simulink model "Maglev_sim_2"  (R2024b)
settings: Solver=ode23tb  StartTime=0.0  StopTime=15  MaxStep=1e-3  RelTol=1e-3
undefined symbols (not defined in the file): A, A0, A0_obv, Adj, B, B0, B0_obv, c, C, C0, C0_obv, D, D0, D0_obv, F, G, K, K0
libraries: simulink x4
settings Model: Creator=coron  LastModifiedBy=rgivo

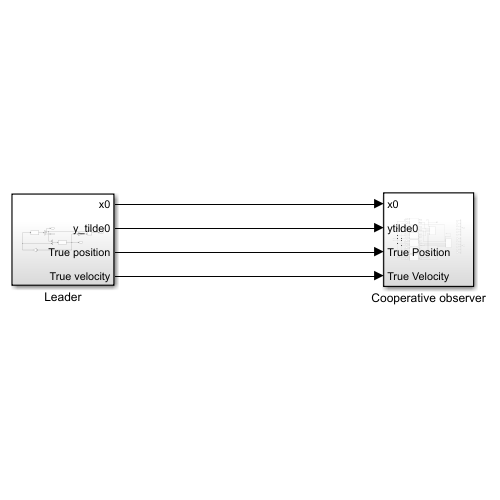
[thumbnail: Simulink's stored preview of the top-level diagram]
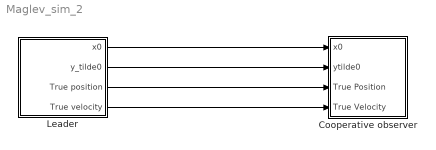
== system Maglev_sim_2 ==
  Cooperative observer : Subsystem
  Leader : Subsystem
  wires:
  Leader/1(x0) -> Cooperative observer/1(x0)
  Leader/2(y_tilde0) -> Cooperative observer/2(ytilde0)
  Leader/3(True position) -> Cooperative observer/3(True Position)
  Leader/4(True velocity) -> Cooperative observer/4(True Velocity)

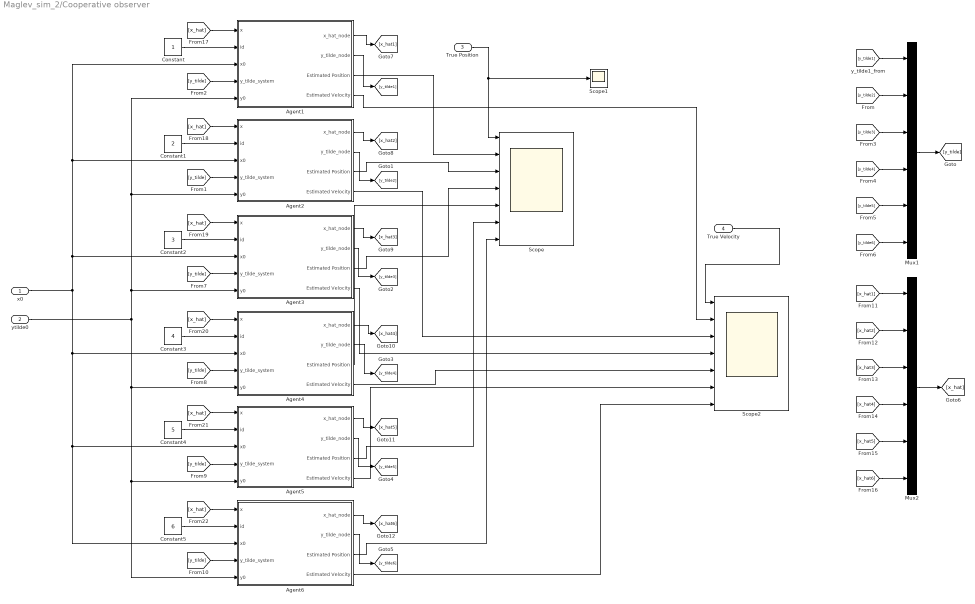
== system Maglev_sim_2/Cooperative observer ==
  x0 : Inport
  ytilde0 : Inport  Port=2
  True Position : Inport  Port=3
  True Velocity : Inport  Port=4
  Agent1 : Subsystem
  Agent2 : Subsystem
  Agent3 : Subsystem
  Agent4 : Subsystem
  Agent5 : Subsystem
  Agent6 : Subsystem
  Constant : Constant
  Constant1 : Constant  Value=2
  Constant2 : Constant  Value=3
  Constant3 : Constant  Value=4
  Constant4 : Constant  Value=5
  Constant5 : Constant  Value=6
  Mux1 : Mux  Inputs=6
  Mux2 : Mux  Inputs=6
  Scope : Scope  NumInputPorts=7
  Scope1 : Scope
  Scope2 : Scope  NumInputPorts=7
  wires:
  Agent4/1(x_hat_node) -> [x_hat4]
  Constant/1 -> Agent1/2(id)
  Constant5/1 -> Agent6/2(id)
  Constant2/1 -> Agent3/2(id)
  Agent2/1(x_hat_node) -> [x_hat2]
  Constant3/1 -> Agent4/2(id)
  Agent5/1(x_hat_node) -> [x_hat5]
  Constant1/1 -> Agent2/2(id)
  Agent3/1(x_hat_node) -> [x_hat3]
  Constant4/1 -> Agent5/2(id)
  Agent1/2(y_tilde_node) -> [y_tilde1]
  [y_tilde1] -> Mux1/1
  Mux1/1 -> [y_tilde]
  Agent2/2(y_tilde_node) -> [y_tilde2]
  [y_tilde2] -> Mux1/2
  [y_tilde] -> Agent2/4(y_tilde_system)
  [y_tilde] -> Agent1/4(y_tilde_system)
  Agent3/2(y_tilde_node) -> [y_tilde3]
  [y_tilde3] -> Mux1/3
  Agent4/2(y_tilde_node) -> [y_tilde4]
  Agent5/2(y_tilde_node) -> [y_tilde5]
  Agent6/2(y_tilde_node) -> [y_tilde6]
  [y_tilde4] -> Mux1/4
  [y_tilde5] -> Mux1/5
  [y_tilde6] -> Mux1/6
  [y_tilde] -> Agent3/4(y_tilde_system)
  [y_tilde] -> Agent4/4(y_tilde_system)
  [y_tilde] -> Agent5/4(y_tilde_system)
  [y_tilde] -> Agent6/4(y_tilde_system)
  Mux2/1 -> [x_hat]
  [x_hat6] -> Mux2/6
  [x_hat5] -> Mux2/5
  [x_hat4] -> Mux2/4
  [x_hat3] -> Mux2/3
  [x_hat2] -> Mux2/2
  [x_hat] -> Agent1/1(x)
  [x_hat] -> Agent2/1(x)
  [x_hat] -> Agent3/1(x)
  [x_hat] -> Agent4/1(x)
  [x_hat] -> Agent5/1(x)
  [x_hat] -> Agent6/1(x)
  ytilde0/1 -> Agent1/5(y0), Agent2/5(y0), Agent3/5(y0), Agent5/5(y0), Agent6/5(y0), Agent4/5(y0)
  x0/1 -> Agent1/3(x0), Agent2/3(x0), Agent3/3(x0), Agent5/3(x0), Agent6/3(x0), Agent4/3(x0)
  Agent6/1(x_hat_node) -> [x_hat6]
  Agent1/1(x_hat_node) -> [x_hat1]
  [x_hat1] -> Mux2/1
  True Position/1 -> Scope/1, Scope1/1
  Agent1/3(Estimated Position) -> Scope/2
  True Velocity/1 -> Scope2/1
  Agent1/4(Estimated Velocity) -> Scope2/2
  Agent2/3(Estimated Position) -> Scope/3
  Agent3/3(Estimated Position) -> Scope/4
  Agent4/3(Estimated Position) -> Scope/5
  Agent5/3(Estimated Position) -> Scope/6
  Agent6/3(Estimated Position) -> Scope/7
  Agent2/4(Estimated Velocity) -> Scope2/3
  Agent3/4(Estimated Velocity) -> Scope2/4
  Agent4/4(Estimated Velocity) -> Scope2/5
  Agent5/4(Estimated Velocity) -> Scope2/6
  Agent6/4(Estimated Velocity) -> Scope2/7

== system Maglev_sim_2/Leader ==
  Add1 : Sum  Inputs=+-
  Demux : Demux  Outputs=3
  Gain1 : Gain  Gain=-K0  Multiplication=Matrix(K*u)
  Gain2 : Gain  Gain=C  Multiplication=Matrix(K*u)
  Luenberger Observer1 : StateSpace  A=A0_obv  B=B0_obv  C=C0_obv  D=D0_obv  InitialCondition=0
  Maglev1 : StateSpace  A=A0  B=B0  C=C0  D=D0  InitialCondition=[0 10]'
  Mux3 : Mux  Inputs=2
  x0 : Outport
  y_tilde0 : Outport  Port=2
  True position : Outport  Port=3
  True velocity : Outport  Port=4
  wires:
  Luenberger Observer1/1 -> Gain2/1, x0/1, Gain1/1
  Mux3/1 -> Luenberger Observer1/1
  Demux/1 -> Mux3/1, Add1/1  "y"
  Demux/3 -> True velocity/1
  Demux/2 -> True position/1
  Maglev1/1 -> Demux/1
  Gain1/1 -> Maglev1/1, Mux3/2  "u = -K*x"
  Gain2/1 -> Add1/2
  Add1/1 -> y_tilde0/1

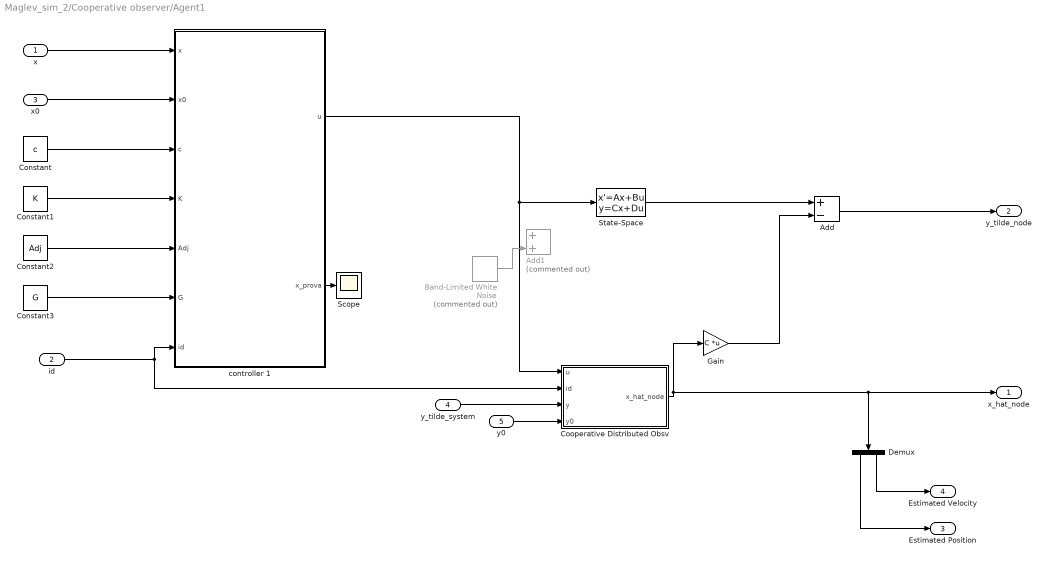
== system Maglev_sim_2/Cooperative observer/Agent1 ==
  x : Inport
  id : Inport  Port=2
  x0 : Inport  Port=3
  y_tilde_system : Inport  Port=4
  y0 : Inport  Port=5
  Add : Sum  Inputs=+-
  Add1 : Sum  Commented=on
  Band-Limited White Noise : simulink/Sources/Band-Limited White Noise  Commented=on  Cov=[0.1]  Ts=0.1  seed=[23341]
  Constant : Constant  Value=c
  Constant1 : Constant  Value=K  VectorParams1D=off
  Constant2 : Constant  Value=Adj
  Constant3 : Constant  Value=G
  Cooperative Distributed Obsv : Subsystem
  Demux : Demux  Outputs=2
  Gain : Gain  Gain=C  Multiplication=Matrix(K*u)
  Scope : Scope
  State-Space : StateSpace  A=(A-B*K0)  B=B  C=C  D=D  InitialCondition=0
  controller 1 : MATLAB Function  TreatAsAtomicUnit=on
  x_hat_node : Outport
  y_tilde_node : Outport  Port=2
  Estimated Position : Outport  Port=3
  Estimated Velocity : Outport  Port=4
  wires:
  x/1 -> controller 1/1(x)
  Constant/1 -> controller 1/3(c)
  Constant1/1 -> controller 1/4(K)
  Constant2/1 -> controller 1/5(Adj)
  Constant3/1 -> controller 1/6(G)
  id/1 -> Cooperative Distributed Obsv/2(id), controller 1/7(id)
  controller 1/1(u) -> Cooperative Distributed Obsv/1(u), State-Space/1
  x0/1 -> controller 1/2(x0)
  controller 1/2(x_prova) -> Scope/1
  y_tilde_system/1 -> Cooperative Distributed Obsv/3(y)
  Cooperative Distributed Obsv/1(x_hat_node) -> Gain/1, Demux/1, x_hat_node/1
  Gain/1 -> Add/2
  State-Space/1 -> Add/1
  Add/1 -> y_tilde_node/1
  Band-Limited White Noise/1 -> Add1/2
  y0/1 -> Cooperative Distributed Obsv/4(y0)
  Demux/1 -> Estimated Position/1
  Demux/2 -> Estimated Velocity/1

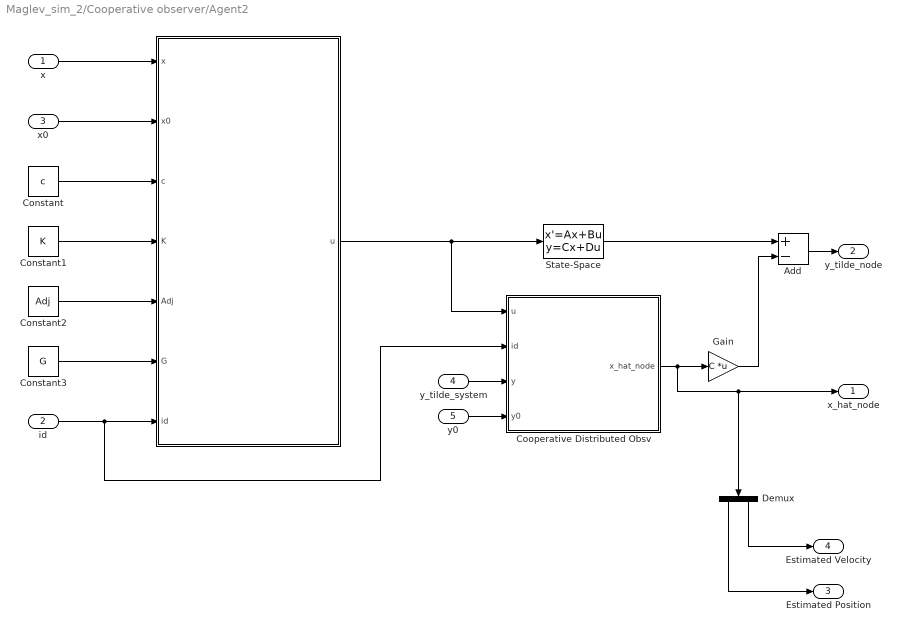
== system Maglev_sim_2/Cooperative observer/Agent2 ==
  x : Inport
  id : Inport  Port=2
  x0 : Inport  Port=3
  y_tilde_system : Inport  Port=4
  y0 : Inport  Port=5
  " " : MATLAB Function  TreatAsAtomicUnit=on
  Add : Sum  Inputs=+-
  Constant : Constant  Value=c
  Constant1 : Constant  Value=K  VectorParams1D=off
  Constant2 : Constant  Value=Adj  VectorParams1D=off
  Constant3 : Constant  Value=G
  Cooperative Distributed Obsv : Subsystem
  Demux : Demux  Outputs=2
  Gain : Gain  Gain=C  Multiplication=Matrix(K*u)
  State-Space : StateSpace  A=(A-B*K0)  B=B  C=C  D=D  InitialCondition=0
  x_hat_node : Outport
  y_tilde_node : Outport  Port=2
  Estimated Position : Outport  Port=3
  Estimated Velocity : Outport  Port=4
  wires:
  id/1 -> Cooperative Distributed Obsv/2(id), " "/7(id)
  Constant2/1 -> " "/5(Adj)
  x0/1 -> " "/2(x0)
  Constant3/1 -> " "/6(G)
  Constant1/1 -> " "/4(K)
  Constant/1 -> " "/3(c)
  Add/1 -> y_tilde_node/1
  " "/1(u) -> State-Space/1, Cooperative Distributed Obsv/1(u)
  y0/1 -> Cooperative Distributed Obsv/4(y0)
  Gain/1 -> Add/2
  State-Space/1 -> Add/1
  x/1 -> " "/1(x)
  y_tilde_system/1 -> Cooperative Distributed Obsv/3(y)
  Cooperative Distributed Obsv/1(x_hat_node) -> Gain/1, Demux/1, x_hat_node/1
  Demux/1 -> Estimated Position/1
  Demux/2 -> Estimated Velocity/1

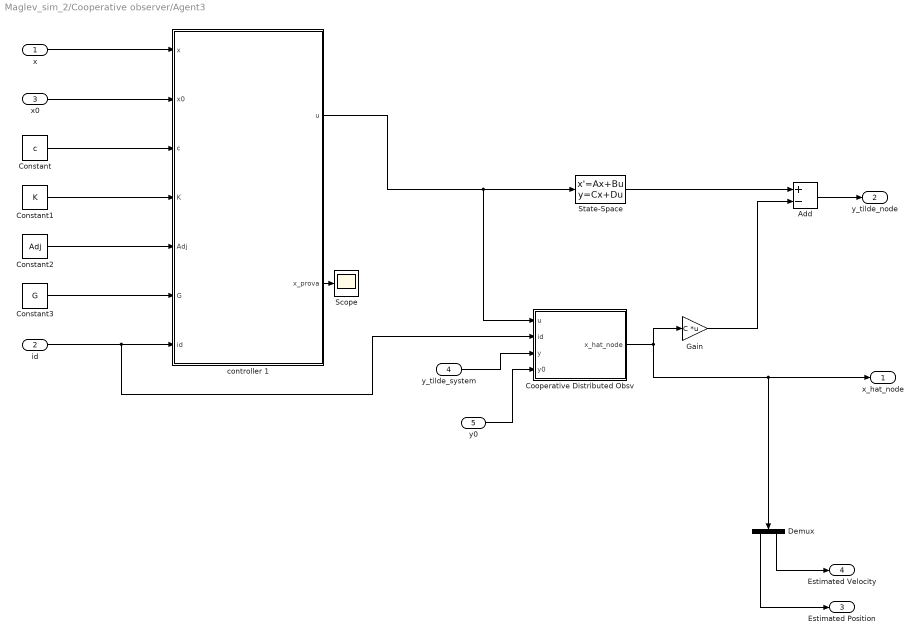
== system Maglev_sim_2/Cooperative observer/Agent3 ==
  x : Inport
  id : Inport  Port=2
  x0 : Inport  Port=3
  y_tilde_system : Inport  Port=4
  y0 : Inport  Port=5
  Add : Sum  Inputs=+-
  Constant : Constant  Value=c
  Constant1 : Constant  Value=K  VectorParams1D=off
  Constant2 : Constant  Value=Adj
  Constant3 : Constant  Value=G
  Cooperative Distributed Obsv : Subsystem
  Demux : Demux  Outputs=2
  Gain : Gain  Gain=C  Multiplication=Matrix(K*u)
  Scope : Scope
  State-Space : StateSpace  A=(A-B*K0)  B=B  C=C  D=D  InitialCondition=0
  controller 1 : MATLAB Function  TreatAsAtomicUnit=on
  x_hat_node : Outport
  y_tilde_node : Outport  Port=2
  Estimated Position : Outport  Port=3
  Estimated Velocity : Outport  Port=4
  wires:
  x/1 -> controller 1/1(x)
  State-Space/1 -> Add/1
  Gain/1 -> Add/2
  controller 1/1(u) -> Cooperative Distributed Obsv/1(u), State-Space/1
  id/1 -> Cooperative Distributed Obsv/2(id), controller 1/7(id)
  Constant2/1 -> controller 1/5(Adj)
  Constant/1 -> controller 1/3(c)
  y0/1 -> Cooperative Distributed Obsv/4(y0)
  Constant1/1 -> controller 1/4(K)
  Add/1 -> y_tilde_node/1
  controller 1/2(x_prova) -> Scope/1
  Constant3/1 -> controller 1/6(G)
  x0/1 -> controller 1/2(x0)
  y_tilde_system/1 -> Cooperative Distributed Obsv/3(y)
  Cooperative Distributed Obsv/1(x_hat_node) -> Demux/1, x_hat_node/1, Gain/1
  Demux/1 -> Estimated Position/1
  Demux/2 -> Estimated Velocity/1

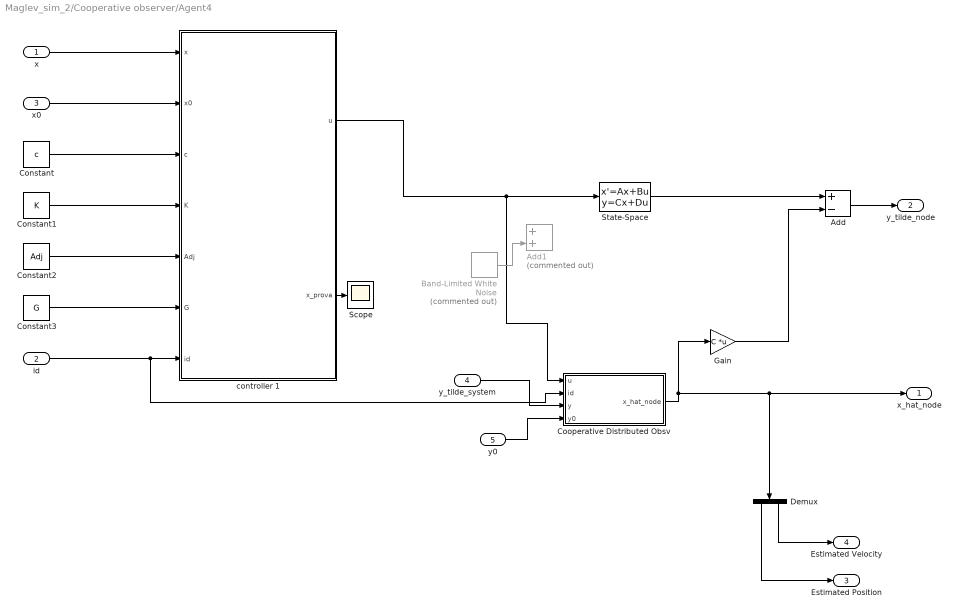
== system Maglev_sim_2/Cooperative observer/Agent4 ==
  x : Inport
  id : Inport  Port=2
  x0 : Inport  Port=3
  y_tilde_system : Inport  Port=4
  y0 : Inport  Port=5
  Add : Sum  Inputs=+-
  Add1 : Sum  Commented=on
  Band-Limited White Noise : simulink/Sources/Band-Limited White Noise  Commented=on  Cov=[0.1]  Ts=0.1  seed=[23341]
  Constant : Constant  Value=c
  Constant1 : Constant  Value=K  VectorParams1D=off
  Constant2 : Constant  Value=Adj
  Constant3 : Constant  Value=G
  Cooperative Distributed Obsv : Subsystem
  Demux : Demux  Outputs=2
  Gain : Gain  Gain=C  Multiplication=Matrix(K*u)
  Scope : Scope
  State-Space : StateSpace  A=(A-B*K0)  B=B  C=C  D=D  InitialCondition=0
  controller 1 : MATLAB Function  TreatAsAtomicUnit=on
  x_hat_node : Outport
  y_tilde_node : Outport  Port=2
  Estimated Position : Outport  Port=3
  Estimated Velocity : Outport  Port=4
  wires:
  x/1 -> controller 1/1(x)
  State-Space/1 -> Add/1
  Gain/1 -> Add/2
  controller 1/1(u) -> Cooperative Distributed Obsv/1(u), State-Space/1
  id/1 -> Cooperative Distributed Obsv/2(id), controller 1/7(id)
  Constant2/1 -> controller 1/5(Adj)
  Constant/1 -> controller 1/3(c)
  y0/1 -> Cooperative Distributed Obsv/4(y0)
  Constant1/1 -> controller 1/4(K)
  Add/1 -> y_tilde_node/1
  Band-Limited White Noise/1 -> Add1/2
  controller 1/2(x_prova) -> Scope/1
  Constant3/1 -> controller 1/6(G)
  x0/1 -> controller 1/2(x0)
  y_tilde_system/1 -> Cooperative Distributed Obsv/3(y)
  Cooperative Distributed Obsv/1(x_hat_node) -> Demux/1, x_hat_node/1, Gain/1
  Demux/1 -> Estimated Position/1
  Demux/2 -> Estimated Velocity/1

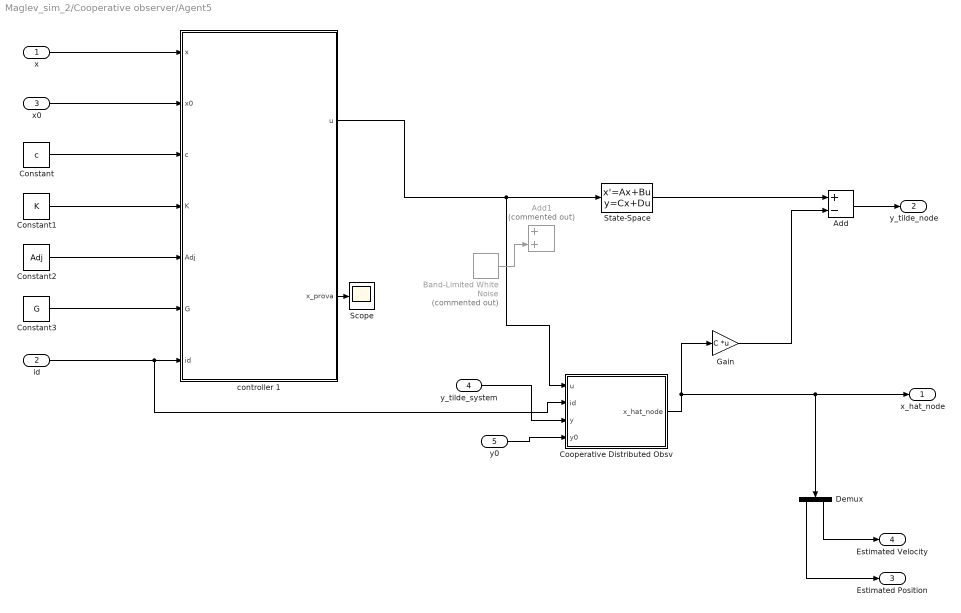
== system Maglev_sim_2/Cooperative observer/Agent5 ==
  x : Inport
  id : Inport  Port=2
  x0 : Inport  Port=3
  y_tilde_system : Inport  Port=4
  y0 : Inport  Port=5
  Add : Sum  Inputs=+-
  Add1 : Sum  Commented=on
  Band-Limited White Noise : simulink/Sources/Band-Limited White Noise  Commented=on  Cov=[0.1]  Ts=0.1  seed=[23341]
  Constant : Constant  Value=c
  Constant1 : Constant  Value=K  VectorParams1D=off
  Constant2 : Constant  Value=Adj
  Constant3 : Constant  Value=G
  Cooperative Distributed Obsv : Subsystem
  Demux : Demux  Outputs=2
  Gain : Gain  Gain=C  Multiplication=Matrix(K*u)
  Scope : Scope
  State-Space : StateSpace  A=(A-B*K0)  B=B  C=C  D=D  InitialCondition=0
  controller 1 : MATLAB Function  TreatAsAtomicUnit=on
  x_hat_node : Outport
  y_tilde_node : Outport  Port=2
  Estimated Position : Outport  Port=3
  Estimated Velocity : Outport  Port=4
  wires:
  x/1 -> controller 1/1(x)
  State-Space/1 -> Add/1
  Gain/1 -> Add/2
  controller 1/1(u) -> Cooperative Distributed Obsv/1(u), State-Space/1
  id/1 -> Cooperative Distributed Obsv/2(id), controller 1/7(id)
  Constant2/1 -> controller 1/5(Adj)
  Constant/1 -> controller 1/3(c)
  y0/1 -> Cooperative Distributed Obsv/4(y0)
  Constant1/1 -> controller 1/4(K)
  Add/1 -> y_tilde_node/1
  Band-Limited White Noise/1 -> Add1/2
  controller 1/2(x_prova) -> Scope/1
  Constant3/1 -> controller 1/6(G)
  x0/1 -> controller 1/2(x0)
  y_tilde_system/1 -> Cooperative Distributed Obsv/3(y)
  Cooperative Distributed Obsv/1(x_hat_node) -> Demux/1, x_hat_node/1, Gain/1
  Demux/1 -> Estimated Position/1
  Demux/2 -> Estimated Velocity/1

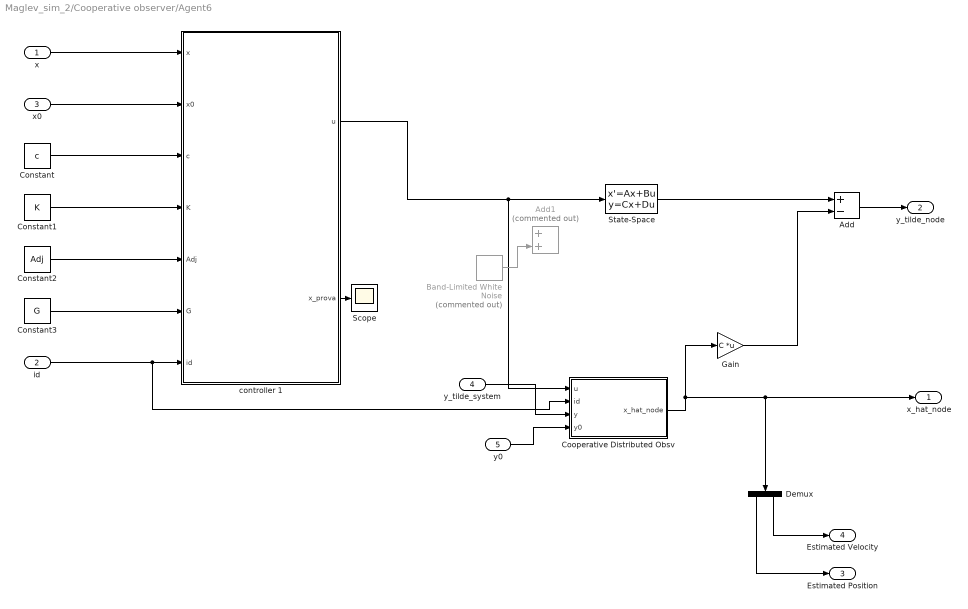
== system Maglev_sim_2/Cooperative observer/Agent6 ==
  x : Inport
  id : Inport  Port=2
  x0 : Inport  Port=3
  y_tilde_system : Inport  Port=4
  y0 : Inport  Port=5
  Add : Sum  Inputs=+-
  Add1 : Sum  Commented=on
  Band-Limited White Noise : simulink/Sources/Band-Limited White Noise  Commented=on  Cov=[0.1]  Ts=0.1  seed=[23341]
  Constant : Constant  Value=c
  Constant1 : Constant  Value=K  VectorParams1D=off
  Constant2 : Constant  Value=Adj
  Constant3 : Constant  Value=G
  Cooperative Distributed Obsv : Subsystem
  Demux : Demux  Outputs=2
  Gain : Gain  Gain=C  Multiplication=Matrix(K*u)
  Scope : Scope
  State-Space : StateSpace  A=(A-B*K0)  B=B  C=C  D=D  InitialCondition=0
  controller 1 : MATLAB Function  TreatAsAtomicUnit=on
  x_hat_node : Outport
  y_tilde_node : Outport  Port=2
  Estimated Position : Outport  Port=3
  Estimated Velocity : Outport  Port=4
  wires:
  x/1 -> controller 1/1(x)
  State-Space/1 -> Add/1
  Gain/1 -> Add/2
  controller 1/1(u) -> Cooperative Distributed Obsv/1(u), State-Space/1
  id/1 -> Cooperative Distributed Obsv/2(id), controller 1/7(id)
  Constant2/1 -> controller 1/5(Adj)
  Constant/1 -> controller 1/3(c)
  y0/1 -> Cooperative Distributed Obsv/4(y0)
  Constant1/1 -> controller 1/4(K)
  Add/1 -> y_tilde_node/1
  Band-Limited White Noise/1 -> Add1/2
  controller 1/2(x_prova) -> Scope/1
  Constant3/1 -> controller 1/6(G)
  x0/1 -> controller 1/2(x0)
  y_tilde_system/1 -> Cooperative Distributed Obsv/3(y)
  Cooperative Distributed Obsv/1(x_hat_node) -> Demux/1, x_hat_node/1, Gain/1
  Demux/1 -> Estimated Position/1
  Demux/2 -> Estimated Velocity/1

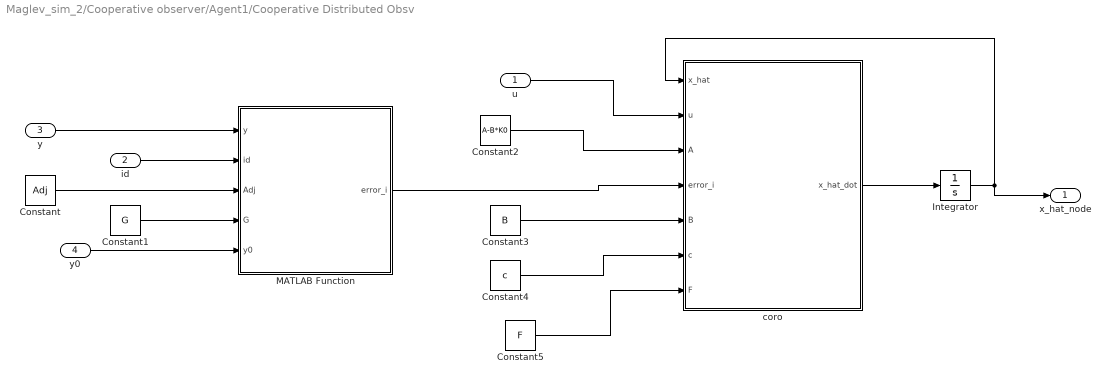
== system Maglev_sim_2/Cooperative observer/Agent1/Cooperative Distributed Obsv ==
  u : Inport
  id : Inport  Port=2
  y : Inport  Port=3
  y0 : Inport  Port=4
  Constant : Constant  Value=Adj
  Constant1 : Constant  Value=G
  Constant2 : Constant  Value=A-B*K0
  Constant3 : Constant  Value=B
  Constant4 : Constant  Value=c
  Constant5 : Constant  Value=F  VectorParams1D=off
  Integrator : Integrator
  MATLAB Function : MATLAB Function  TreatAsAtomicUnit=on
  coro : MATLAB Function  TreatAsAtomicUnit=on
  x_hat_node : Outport
  wires:
  id/1 -> MATLAB Function/2(id)
  Constant/1 -> MATLAB Function/3(Adj)
  Constant1/1 -> MATLAB Function/4(G)
  u/1 -> coro/2(u)
  MATLAB Function/1(error_i) -> coro/4(error_i)
  Constant2/1 -> coro/3(A)
  Constant3/1 -> coro/5(B)
  Constant4/1 -> coro/6(c)
  Constant5/1 -> coro/7(F)
  coro/1(x_hat_dot) -> Integrator/1
  Integrator/1 -> x_hat_node/1, coro/1(x_hat)
  y0/1 -> MATLAB Function/5(y0)
  y/1 -> MATLAB Function/1(y)

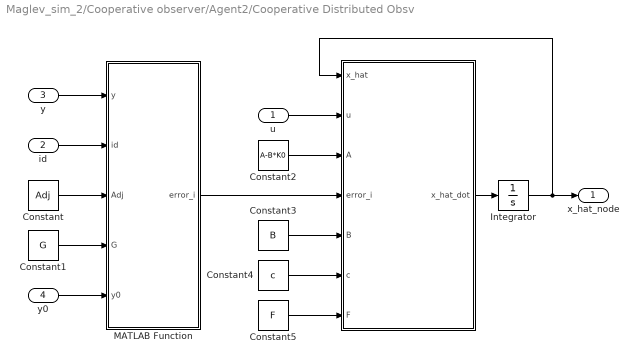
== system Maglev_sim_2/Cooperative observer/Agent2/Cooperative Distributed Obsv ==
  u : Inport
  id : Inport  Port=2
  y : Inport  Port=3
  y0 : Inport  Port=4
  " " : MATLAB Function  TreatAsAtomicUnit=on
  Constant : Constant  Value=Adj
  Constant1 : Constant  Value=G
  Constant2 : Constant  Value=A-B*K0
  Constant3 : Constant  Value=B
  Constant4 : Constant  Value=c
  Constant5 : Constant  Value=F  VectorParams1D=off
  Integrator : Integrator
  MATLAB Function : MATLAB Function  TreatAsAtomicUnit=on
  x_hat_node : Outport
  wires:
  Constant/1 -> MATLAB Function/3(Adj)
  Integrator/1 -> x_hat_node/1, " "/1(x_hat)
  MATLAB Function/1(error_i) -> " "/4(error_i)
  " "/1(x_hat_dot) -> Integrator/1
  Constant2/1 -> " "/3(A)
  y/1 -> MATLAB Function/1(y)
  Constant4/1 -> " "/6(c)
  u/1 -> " "/2(u)
  Constant5/1 -> " "/7(F)
  y0/1 -> MATLAB Function/5(y0)
  id/1 -> MATLAB Function/2(id)
  Constant3/1 -> " "/5(B)
  Constant1/1 -> MATLAB Function/4(G)

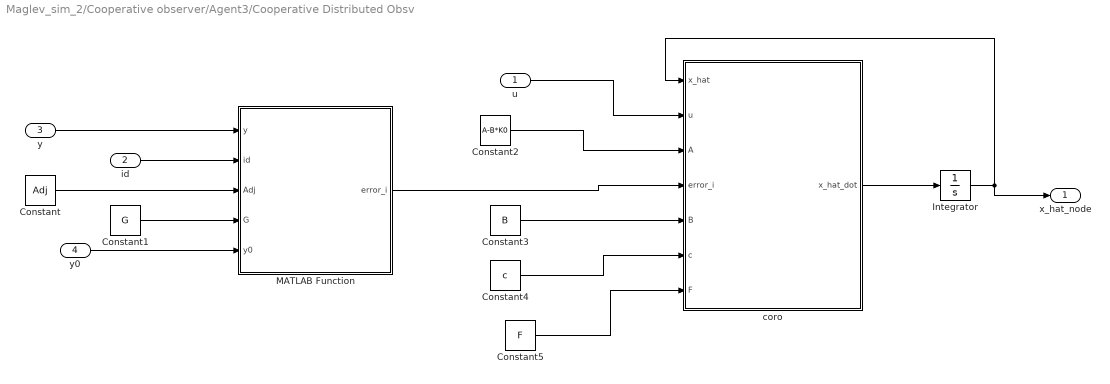
== system Maglev_sim_2/Cooperative observer/Agent3/Cooperative Distributed Obsv ==
  u : Inport
  id : Inport  Port=2
  y : Inport  Port=3
  y0 : Inport  Port=4
  Constant : Constant  Value=Adj
  Constant1 : Constant  Value=G
  Constant2 : Constant  Value=A-B*K0
  Constant3 : Constant  Value=B
  Constant4 : Constant  Value=c
  Constant5 : Constant  Value=F  VectorParams1D=off
  Integrator : Integrator
  MATLAB Function : MATLAB Function  TreatAsAtomicUnit=on
  coro : MATLAB Function  TreatAsAtomicUnit=on
  x_hat_node : Outport
  wires:
  Constant/1 -> MATLAB Function/3(Adj)
  Integrator/1 -> x_hat_node/1, coro/1(x_hat)
  MATLAB Function/1(error_i) -> coro/4(error_i)
  coro/1(x_hat_dot) -> Integrator/1
  Constant2/1 -> coro/3(A)
  y/1 -> MATLAB Function/1(y)
  Constant4/1 -> coro/6(c)
  u/1 -> coro/2(u)
  Constant5/1 -> coro/7(F)
  y0/1 -> MATLAB Function/5(y0)
  id/1 -> MATLAB Function/2(id)
  Constant3/1 -> coro/5(B)
  Constant1/1 -> MATLAB Function/4(G)

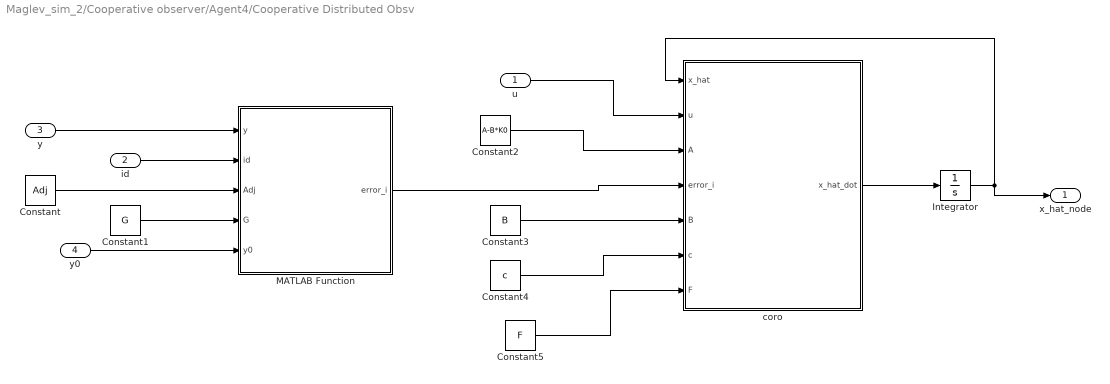
== system Maglev_sim_2/Cooperative observer/Agent4/Cooperative Distributed Obsv ==
  u : Inport
  id : Inport  Port=2
  y : Inport  Port=3
  y0 : Inport  Port=4
  Constant : Constant  Value=Adj
  Constant1 : Constant  Value=G
  Constant2 : Constant  Value=A-B*K0
  Constant3 : Constant  Value=B
  Constant4 : Constant  Value=c
  Constant5 : Constant  Value=F  VectorParams1D=off
  Integrator : Integrator
  MATLAB Function : MATLAB Function  TreatAsAtomicUnit=on
  coro : MATLAB Function  TreatAsAtomicUnit=on
  x_hat_node : Outport
  wires:
  Constant/1 -> MATLAB Function/3(Adj)
  Integrator/1 -> x_hat_node/1, coro/1(x_hat)
  MATLAB Function/1(error_i) -> coro/4(error_i)
  coro/1(x_hat_dot) -> Integrator/1
  Constant2/1 -> coro/3(A)
  y/1 -> MATLAB Function/1(y)
  Constant4/1 -> coro/6(c)
  u/1 -> coro/2(u)
  Constant5/1 -> coro/7(F)
  y0/1 -> MATLAB Function/5(y0)
  id/1 -> MATLAB Function/2(id)
  Constant3/1 -> coro/5(B)
  Constant1/1 -> MATLAB Function/4(G)

== system Maglev_sim_2/Cooperative observer/Agent5/Cooperative Distributed Obsv ==
  u : Inport
  id : Inport  Port=2
  y : Inport  Port=3
  y0 : Inport  Port=4
  Constant : Constant  Value=Adj
  Constant1 : Constant  Value=G
  Constant2 : Constant  Value=A-B*K0
  Constant3 : Constant  Value=B
  Constant4 : Constant  Value=c
  Constant5 : Constant  Value=F  VectorParams1D=off
  Integrator : Integrator
  MATLAB Function : MATLAB Function  TreatAsAtomicUnit=on
  coro : MATLAB Function  TreatAsAtomicUnit=on
  x_hat_node : Outport
  wires:
  Constant/1 -> MATLAB Function/3(Adj)
  Integrator/1 -> x_hat_node/1, coro/1(x_hat)
  MATLAB Function/1(error_i) -> coro/4(error_i)
  coro/1(x_hat_dot) -> Integrator/1
  Constant2/1 -> coro/3(A)
  y/1 -> MATLAB Function/1(y)
  Constant4/1 -> coro/6(c)
  u/1 -> coro/2(u)
  Constant5/1 -> coro/7(F)
  y0/1 -> MATLAB Function/5(y0)
  id/1 -> MATLAB Function/2(id)
  Constant3/1 -> coro/5(B)
  Constant1/1 -> MATLAB Function/4(G)

== system Maglev_sim_2/Cooperative observer/Agent6/Cooperative Distributed Obsv ==
  u : Inport
  id : Inport  Port=2
  y : Inport  Port=3
  y0 : Inport  Port=4
  Constant : Constant  Value=Adj
  Constant1 : Constant  Value=G
  Constant2 : Constant  Value=A-B*K0
  Constant3 : Constant  Value=B
  Constant4 : Constant  Value=c
  Constant5 : Constant  Value=F  VectorParams1D=off
  Integrator : Integrator
  MATLAB Function : MATLAB Function  TreatAsAtomicUnit=on
  coro : MATLAB Function  TreatAsAtomicUnit=on
  x_hat_node : Outport
  wires:
  Constant/1 -> MATLAB Function/3(Adj)
  y/1 -> MATLAB Function/1(y)
  Constant4/1 -> coro/6(c)
  u/1 -> coro/2(u)
  MATLAB Function/1(error_i) -> coro/4(error_i)
  Integrator/1 -> x_hat_node/1, coro/1(x_hat)
  Constant5/1 -> coro/7(F)
  Constant1/1 -> MATLAB Function/4(G)
  id/1 -> MATLAB Function/2(id)
  Constant2/1 -> coro/3(A)
  Constant3/1 -> coro/5(B)
  y0/1 -> MATLAB Function/5(y0)
  coro/1(x_hat_dot) -> Integrator/1

== matlab function Maglev_sim_2/Cooperative observer/Agent2/Cooperative Distributed Obsv/  ==
  data: x_hat input; u input; x_hat_dot output; A input; error_i input; B input; c input; F input
function x_hat_dot = fcn(x_hat,u,A,error_i,B,c,F)

x_hat_dot = A*x_hat + B*u - c*F*error_i;

== matlab function Maglev_sim_2/Cooperative observer/Agent2/  ==
  data: x input; x0 input; u output; c input; K input; Adj input; G input; id input
function u = controller(x,x0,c,K,Adj,G,id)


pairs = reshape(x, 2, [])';

error = zeros(2,1);

for j = 1:6
    error = error + Adj(id,j)*(pairs(j,:)'-pairs(id,:)')+G(id)*(x0 - pairs(id,:)');
end
u=c*K*error;

== matlab function Maglev_sim_2/Cooperative observer/Agent3/Cooperative Distributed Obsv/coro ==
  data: x_hat input; u input; x_hat_dot output; A input; error_i input; B input; c input; F input
function x_hat_dot = fcn(x_hat,u,A,error_i,B,c,F)

x_hat_dot = A*x_hat + B*u - c*F*error_i;

== matlab function Maglev_sim_2/Cooperative observer/Agent1/controller 1 ==
  data: x input; x0 input; u output; c input; K input; Adj input; G input; id input; x_prova output
function [u,x_prova]= controller(x,x0,c,K,Adj,G,id)


pairs = reshape(x, 2, [])';

error = zeros(2,1);

for j = 1:6
    error = error + Adj(id,j)*(pairs(j,:)'-pairs(id,:)')+G(id)*(x0 - pairs(id,:)');
end

x_prova = pairs(id,:)';

u=c*K*error;

== matlab function Maglev_sim_2/Cooperative observer/Agent3/controller 1 ==
  data: x input; x0 input; u output; c input; K input; Adj input; G input; id input; x_prova output
function [u,x_prova]= controller(x,x0,c,K,Adj,G,id)


pairs = reshape(x, 2, [])';

error = zeros(2,1);

for j = 1:6
    error = error + Adj(id,j)*(pairs(j,:)'-pairs(id,:)')+G(id)*(x0 - pairs(id,:)');
end

x_prova = pairs(id,:)';

u=c*K*error;

== matlab function Maglev_sim_2/Cooperative observer/Agent4/Cooperative Distributed Obsv/coro ==
  data: x_hat input; u input; x_hat_dot output; A input; error_i input; B input; c input; F input
function x_hat_dot = fcn(x_hat,u,A,error_i,B,c,F)

x_hat_dot = A*x_hat + B*u - c*F*error_i;

== matlab function Maglev_sim_2/Cooperative observer/Agent4/controller 1 ==
  data: x input; x0 input; u output; c input; K input; Adj input; G input; id input; x_prova output
function [u,x_prova]= controller(x,x0,c,K,Adj,G,id)


pairs = reshape(x, 2, [])';

error = zeros(2,1);

for j = 1:6
    error = error + Adj(id,j)*(pairs(j,:)'-pairs(id,:)')+G(id)*(x0 - pairs(id,:)');
end

x_prova = pairs(id,:)';

u=c*K*error;

== matlab function Maglev_sim_2/Cooperative observer/Agent5/Cooperative Distributed Obsv/coro ==
  data: x_hat input; u input; x_hat_dot output; A input; error_i input; B input; c input; F input
function x_hat_dot = fcn(x_hat,u,A,error_i,B,c,F)

x_hat_dot = A*x_hat + B*u - c*F*error_i;

== matlab function Maglev_sim_2/Cooperative observer/Agent5/controller 1 ==
  data: x input; x0 input; u output; c input; K input; Adj input; G input; id input; x_prova output
function [u,x_prova]= controller(x,x0,c,K,Adj,G,id)


pairs = reshape(x, 2, [])';

error = zeros(2,1);

for j = 1:6
    error = error + Adj(id,j)*(pairs(j,:)'-pairs(id,:)')+G(id)*(x0 - pairs(id,:)');
end

x_prova = pairs(id,:)';

u=c*K*error;

== matlab function Maglev_sim_2/Cooperative observer/Agent6/Cooperative Distributed Obsv/coro ==
  data: x_hat input; u input; x_hat_dot output; A input; error_i input; B input; c input; F input
function x_hat_dot = fcn(x_hat,u,A,error_i,B,c,F)

x_hat_dot = A*x_hat + B*u - c*F*error_i;

== matlab function Maglev_sim_2/Cooperative observer/Agent6/controller 1 ==
  data: x input; x0 input; u output; c input; K input; Adj input; G input; id input; x_prova output
function [u,x_prova]= controller(x,x0,c,K,Adj,G,id)


pairs = reshape(x, 2, [])';

error = zeros(2,1);

for j = 1:6
    error = error + Adj(id,j)*(pairs(j,:)'-pairs(id,:)')+G(id)*(x0 - pairs(id,:)');
end

x_prova = pairs(id,:)';

u=c*K*error;

== matlab function Maglev_sim_2/Cooperative observer/Agent2/Cooperative Distributed Obsv/MATLAB Function ==
  data: y input; error_i output; id input; Adj input; G input; y0 input
function error_i = fcn(y,id,Adj,G,y0)


error = 0;

%% check y dovrebbe essere 1x1
for j = 1:6
    error = error + Adj(id,j)*(y(j)-y(id))+G(id)*(y0 - y(id));
end

error_i = error;

== matlab function Maglev_sim_2/Cooperative observer/Agent6/Cooperative Distributed Obsv/MATLAB Function ==
  data: y input size=[1 6]; error_i output; id input; Adj input; G input; y0 input
function error_i = fcn(y,id,Adj,G,y0)


error = 0;

%% check y dovrebbe essere 1x1
for j = 1:6
    error = error + Adj(id,j)*(y(j)-y(id))+G(id)*(y0 - y(id));
end

error_i = error;

== matlab function Maglev_sim_2/Cooperative observer/Agent3/Cooperative Distributed Obsv/MATLAB Function ==
  data: y input size=[1 6]; error_i output; id input; Adj input; G input; y0 input
function error_i = fcn(y,id,Adj,G,y0)


error = 0;

%% check y dovrebbe essere 1x1
for j = 1:6
    error = error + Adj(id,j)*(y(j)-y(id))+G(id)*(y0 - y(id));
end

error_i = error;

== matlab function Maglev_sim_2/Cooperative observer/Agent4/Cooperative Distributed Obsv/MATLAB Function ==
  data: y input size=[1 6]; error_i output; id input; Adj input; G input; y0 input
function error_i = fcn(y,id,Adj,G,y0)


error = 0;

%% check y dovrebbe essere 1x1
for j = 1:6
    error = error + Adj(id,j)*(y(j)-y(id))+G(id)*(y0 - y(id));
end

error_i = error;

== matlab function Maglev_sim_2/Cooperative observer/Agent5/Cooperative Distributed Obsv/MATLAB Function ==
  data: y input size=[1 6]; error_i output; id input; Adj input; G input; y0 input
function error_i = fcn(y,id,Adj,G,y0)


error = 0;

%% check y dovrebbe essere 1x1
for j = 1:6
    error = error + Adj(id,j)*(y(j)-y(id))+G(id)*(y0 - y(id));
end

error_i = error;

== matlab function Maglev_sim_2/Cooperative observer/Agent1/Cooperative Distributed Obsv/MATLAB Function ==
  data: y input size=[1 6]; error_i output; id input; Adj input; G input; y0 input
function error_i = fcn(y,id,Adj,G,y0)


error = 0;

%% check y dovrebbe essere 1x1
for j = 1:6
    error = error + Adj(id,j)*(y(j)-y(id))+G(id)*(y0 - y(id));
end

error_i = error;

== matlab function Maglev_sim_2/Cooperative observer/Agent1/Cooperative Distributed Obsv/coro ==
  data: x_hat input; u input; x_hat_dot output; A input; error_i input; B input; c input; F input
function x_hat_dot = fcn(x_hat,u,A,error_i,B,c,F)

x_hat_dot = A*x_hat + B*u - c*F*error_i;
